simulink model "ex2_encoder"  (R2023b)
settings: Solver=FixedStepAuto  StartTime=0.0  StopTime=inf  FixedStep=0.01  RelTol=1e-3
values from neighbouring files (symbols this model uses):
  J = 0.02    [motor_ex.m]    (also in params.m)
  Kb = 0.1    [motor_ex.m]    (also in params.m)
  KD = 0.5    [ex1_pid.m]    (also in params.m)
  Kf = 0.2    [motor_ex.m]    (also in params.m = 0.01)
  KI = 0.1    [ex1_pid.m]    (also in params.m)
  Km = 0.1    [motor_ex.m]    (also in params.m = 1)
  KP = 0.7    [ex1_pid.m]    (also in params.m)
  L = 0.5    [motor_ex.m]    (also in params.m)
  R = 2.0    (= 2)    [motor_ex.m]    (also in params.m)
libraries: arduinolib x4, simulink x1, arduinosensorlib x1
settings Model: ExtModeTrigDuration=2  Creator=SJ  LastModifiedBy=SJ
settings SolverCC: AutoInsertRateTranBlk=on
settings OptimizationCC: EnhancedBackFolding=on  PassReuseOutputArgsAs=Individual arguments  ZeroExternalMemoryAtStartup=off  ZeroInternalMemoryAtStartup=off  MaxStackSize=64  OptimizeBlockOrder=speed  DifferentSizesBufferReuse=on  OptimizationCustomize=off  EfficientTunableParamExpr=on
settings DebuggingCC: MultiTaskRateTransMsg=warning  ParameterTunabilityLossMsg=error
settings HardwareCC: ProdBitPerInt=16  ProdBitPerPointer=16  ProdBitPerSizeT=16  ProdBitPerPtrDiffT=16  ProdLargestAtomicFloat=None  ProdWordSize=8  ProdHWDeviceType=Atmel->AVR
settings SFSimCC: MATLABDynamicMemAlloc=off
settings RTWCC: Description=Embedded Coder  SystemTargetFile=ert.tlc  HardwareBoard=Arduino Mega 2560  TemplateMakefile=ert_default_tmf  Toolchain=Arduino AVR  BuildConfiguration=Faster Runs
settings CodeAppCC: ForceParamTrailComments=on  IgnoreCustomStorageClasses=off  OperatorAnnotations=on  SimulinkDataObjDesc=on  SFDataObjDesc=on  InsertBlockDesc=on
settings ERTTargetCC: SupportContinuousTime=on  SupportVariableSizeSignals=on  ExtModeTransport=3  ExtModeStaticAlloc=on  ExtModeAutomaticAllocSize=off  ExtModeStaticAllocSize=2048  ExtModeMexFile=ext_xcp  ExtModeIntrfLevel=Level2 - Open

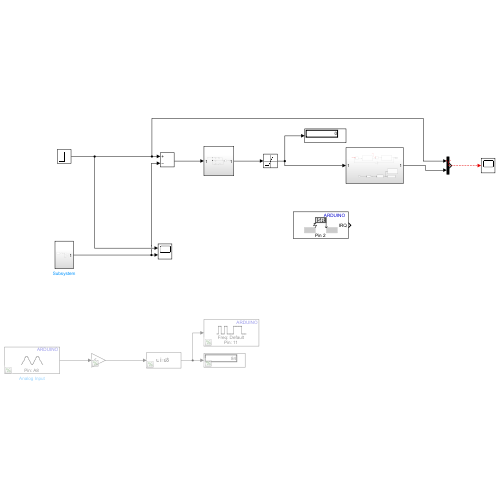
[thumbnail: Simulink's stored preview of the top-level diagram]
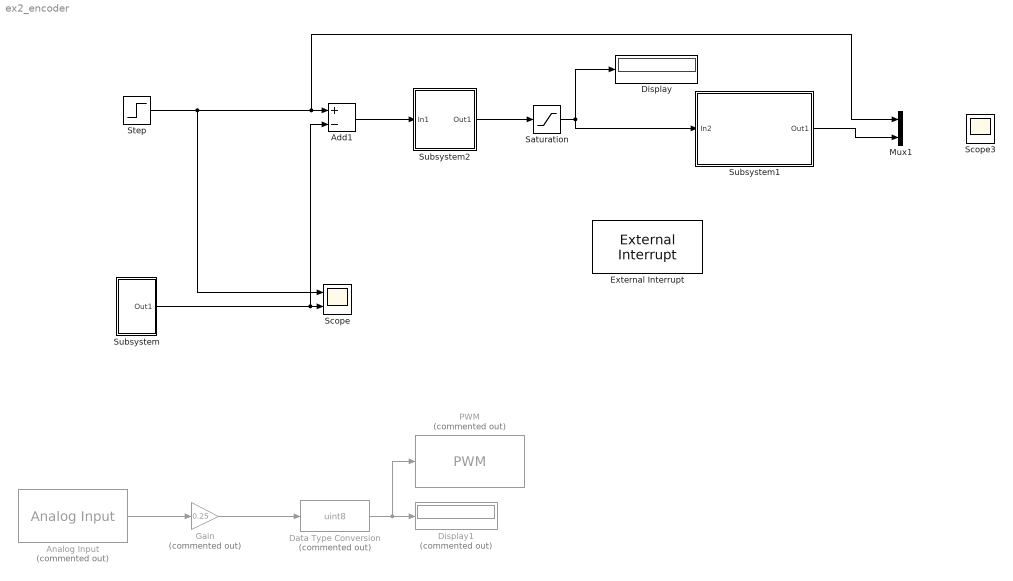
== system ex2_encoder ==
  Add1 : Sum  Inputs=+-
  Analog Input : arduinolib/Analog Input  Commented=on  pinNumber=8  ReadResultsOnly=off  ConversionTriggerSource=Software  ExternalTriggerType=uint32( 0 )  OutputDataType=uint16  EnableConversionCompleteNotify=off  EnableOuputStatus=off  SampleTime=-1  blockPlatform=arduino
  Data Type Conversion : DataTypeConversion  Commented=on  OutDataTypeStr=uint8  SaturateOnIntegerOverflow=off  RndMeth=Floor
  Display : Display
  Display1 : Display  Commented=on
  External Interrupt : arduinolib/External Interrupt  Pin=2  PullUp=off  Mode=RISING  InterruptSimulationInput=off
  Gain : Gain  Commented=on  Gain=0.25
  Mux1 : Mux  Inputs=2
  PWM : arduinolib/PWM  Commented=on  pinNumber=11  frequencyType=Default  desiredFrequency=490.2  achievableFrequency=490.2
  Saturation : Saturate  UpperLimit=12  LowerLimit=0
  Scope : Scope  NumInputPorts=2
  Scope3 : Scope
  Step : Step  After=100  SampleTime=0
  Subsystem : Subsystem
  Subsystem1 : Subsystem
  Subsystem2 : Subsystem
  wires:
  Gain/1 -> Data Type Conversion/1
  Data Type Conversion/1 -> Display1/1, PWM/1
  Analog Input/1 -> Gain/1
  Subsystem/1(Out1) -> Add1/2, Scope/2
  ? -> Scope3/1
  Add1/1 -> Subsystem2/1(In1)
  Subsystem1/1(Out1) -> Mux1/2
  Step/1 -> Mux1/1, Add1/1, Scope/1
  Subsystem2/1(Out1) -> Saturation/1
  Saturation/1 -> Subsystem1/1(In2), Display/1

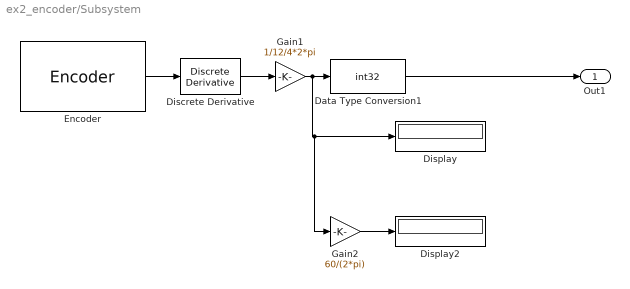
== system ex2_encoder/Subsystem ==
  Data Type Conversion1 : DataTypeConversion  OutDataTypeStr=int32  SaturateOnIntegerOverflow=off  RndMeth=Floor
  Discrete Derivative : simulink/Discrete/Discrete Derivative  gainval=1.0  ICPrevScaledInput=0.0  OutMin=[]  OutMax=[]  OutDataType=fixdt(1, 16)  OutScaling=2^-10  DoSatur=off
  Display : Display
  Display2 : Display
  Encoder : arduinosensorlib/Encoder  InputA=18  InputB=19  Mode=No reset  SampleTime=-1
  Gain1 : Gain  Gain=1/12/4*2*pi
  Gain2 : Gain  Gain=60/(2*pi)
  Out1 : Outport
  wires:
  Gain1/1 -> Gain2/1, Display/1, Data Type Conversion1/1
  Encoder/1 -> Discrete Derivative/1
  Gain2/1 -> Display2/1
  Data Type Conversion1/1 -> Out1/1
  Discrete Derivative/1 -> Gain1/1

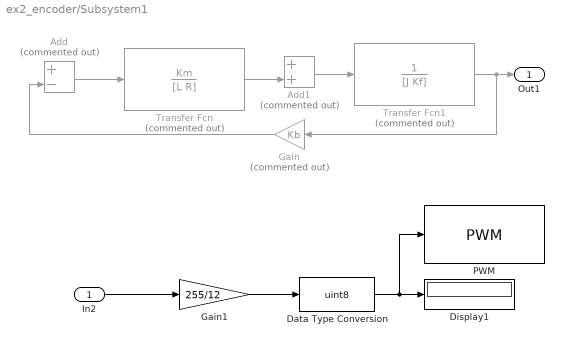
== system ex2_encoder/Subsystem1 ==
  In2 : Inport
  Add : Sum  Commented=on  Inputs=+-
  Add1 : Sum  Commented=on
  Data Type Conversion : DataTypeConversion  OutDataTypeStr=uint8  SaturateOnIntegerOverflow=off  RndMeth=Floor
  Display1 : Display
  Gain : Gain  Commented=on  Gain=Kb
  Gain1 : Gain  Gain=255/12
  PWM : arduinolib/PWM  pinNumber=11  frequencyType=Default  desiredFrequency=490.2  achievableFrequency=490.2
  Transfer Fcn : TransferFcn  Commented=on  Numerator=Km  Denominator=[L R]
  Transfer Fcn1 : TransferFcn  Commented=on  Numerator=1  Denominator=[J Kf]
  Out1 : Outport
  wires:
  ? -> Add/1
  ? -> Add1/1
  Add/1 -> Transfer Fcn/1
  Add1/1 -> Transfer Fcn1/1
  Transfer Fcn/1 -> Add1/2
  Gain/1 -> Add/2
  Transfer Fcn1/1 -> Gain/1, Out1/1
  In2/1 -> Gain1/1
  Gain1/1 -> Data Type Conversion/1
  Data Type Conversion/1 -> Display1/1, PWM/1

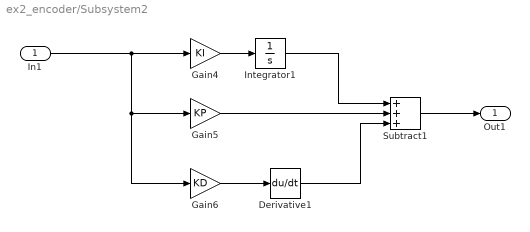
== system ex2_encoder/Subsystem2 ==
  In1 : Inport
  Derivative1 : Derivative
  Gain4 : Gain  Gain=KI
  Gain5 : Gain  Gain=KP
  Gain6 : Gain  Gain=KD
  Integrator1 : Integrator
  Subtract1 : Sum  Inputs=+++
  Out1 : Outport
  wires:
  Subtract1/1 -> Out1/1
  In1/1 -> Gain5/1, Gain6/1, Gain4/1
  Integrator1/1 -> Subtract1/1
  Derivative1/1 -> Subtract1/3
  Gain6/1 -> Derivative1/1
  Gain5/1 -> Subtract1/2
  Gain4/1 -> Integrator1/1
